simulink model "siasun_config_casadi_VS_lsj_robot_16a"  (R2020a)
settings: Solver=FixedStepAuto  StartTime=0.0  StopTime=inf  FixedStep=0.001  RelTol=1e-3  EnableMultiTasking=on
libraries: Robot_ToolBox x20
(part 2 of 6)

== matlab function siasun_config_casadi_VS_lsj_robot_16a/Cartesian_planning_angle/Cartesian_trajectory1 ==
  data: time input; q output; initq output
function [q,initq]  = Cartesian(time)


    %% casadi 优化结果  traj - 6xn

    %% lsj 速度优化结果 traj - 6xn

    % 1/4 Ellipse fast T 2.5201
